simulink model "ddddddddd"  (R2020a)
settings: Solver=VariableStepAuto  StartTime=0.0  StopTime=1  RelTol=1e-3
libraries: powerlib x19, powerlib_meascontrol x4
settings Model: Creator=hp  LastModifiedBy=hp

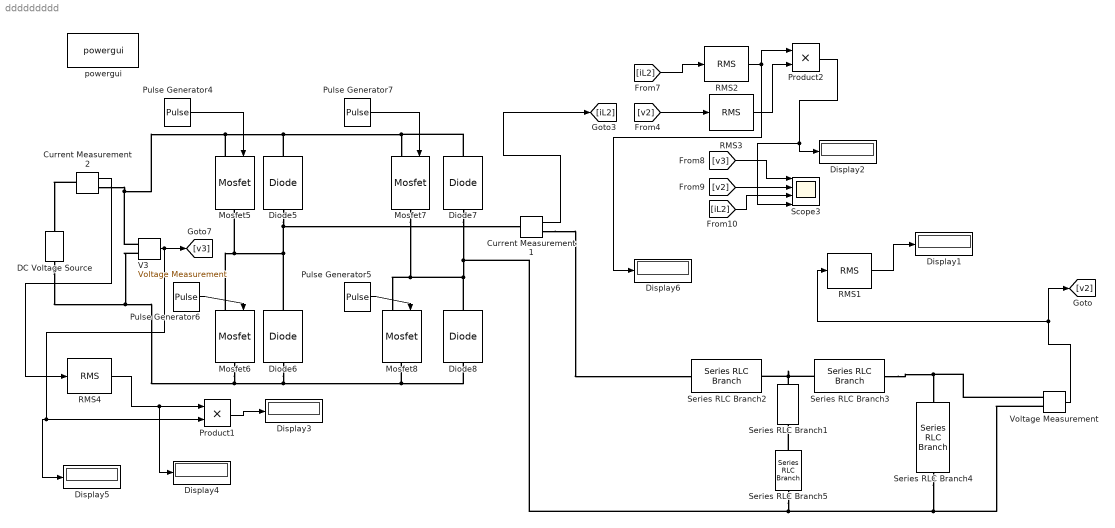
== system ddddddddd ==
  Current Measurement1 : powerlib/Measurements/Current Measurement  PhasorSimulation=off  OutputType=Complex  PSBequivalent=0
  Current Measurement2 : powerlib/Measurements/Current Measurement  PhasorSimulation=off  OutputType=Complex  PSBequivalent=0
  DC Voltage Source : powerlib/Electrical Sources/DC Voltage Source  Amplitude=900  Measurements=None
  Diode{5..8} (4 alike) : powerlib/Power Electronics/Diode  Ron=0.001  Lon=0  Vf=0.8  IC=0  UseSnubber=0  Rs=500  Cs=250e-9  Measurements=off
  Display{1..6} (6 alike) : Display
  Mosfet{5..8} (4 alike) : powerlib/Power Electronics/Mosfet  Ron=0.1  Lon=0  Rd=0.01  Vfd=0  IC=0  Rs=1e5  Cs=inf  Measurements=off
  Product1 : Product
  Product2 : Product
  Pulse Generator4 : DiscretePulseGenerator  PulseType=Time based  Period=1/(10000)  PulseWidth=50  PhaseDelay=0/(360*5000)
  Pulse Generator5 : DiscretePulseGenerator  PulseType=Time based  Period=1/(10000)  PulseWidth=50  PhaseDelay=0/(360*5000)
  Pulse Generator6 : DiscretePulseGenerator  PulseType=Time based  Period=1/(10000)  PulseWidth=50  PhaseDelay=180/(360*10000)
  Pulse Generator7 : DiscretePulseGenerator  PulseType=Time based  Period=1/(10000)  PulseWidth=50  PhaseDelay=180/(360*10000)
  RMS{1..4} (4 alike) : powerlib_meascontrol/Measurements/RMS  TrueRMS=on  Freq=60  RMSInit=120  Ts=0
  Scope3 : Scope  NumInputPorts=4
  Series RLC Branch1 : powerlib/Elements/Series RLC Branch  LConnTagsString=__new0  RConnTagsString=__new0  BranchType=C  Resistance=181  Inductance=1e-3  SetiL0=off  InitialCurrent=0  Capacitance=1.5e-5  Setx0=off  InitialVoltage=0  Measurements=None
  Series RLC Branch2 : powerlib/Elements/Series RLC Branch  LConnTagsString=__new0  RConnTagsString=__new0  BranchType=RL  Resistance=1e-3  Inductance=10e-4  SetiL0=off  InitialCurrent=0  Capacitance=1e-6  Setx0=off  InitialVoltage=0  Measurements=None
  Series RLC Branch3 : powerlib/Elements/Series RLC Branch  LConnTagsString=__new0  RConnTagsString=__new0  BranchType=RL  Resistance=1e-3  Inductance=11e-4  SetiL0=off  InitialCurrent=0  Capacitance=1e-6  Setx0=off  InitialVoltage=0  Measurements=None
  Series RLC Branch4 : powerlib/Elements/Series RLC Branch  LConnTagsString=__new0  RConnTagsString=__new0  BranchType=R  Resistance=181  Inductance=1e-3  SetiL0=off  InitialCurrent=0  Capacitance=1e-6  Setx0=off  InitialVoltage=0  Measurements=None
  Series RLC Branch5 : powerlib/Elements/Series RLC Branch  LConnTagsString=__new0  RConnTagsString=__new0  BranchType=R  Resistance=22.15  Inductance=1e-3  SetiL0=off  InitialCurrent=0  Capacitance=1e-6  Setx0=off  InitialVoltage=0  Measurements=None
  V3 : powerlib/Measurements/Voltage Measurement  PhasorSimulation=off  OutputType=Complex  PSBequivalent=0
  Voltage Measurement : powerlib/Measurements/Voltage Measurement  PhasorSimulation=off  OutputType=Complex  PSBequivalent=0
  powergui : powerlib/powergui  Priority=1  SimulationMode=Discrete  SampleTime=50e-8  frequency=60  Iterations=50  frequencyindice=0  Pbase=100e6  ErrMax=1e-4  UnitsV=kV  UnitsW=MW  buscounter=0  FunctionMessages=off  echomessages=off  EnableUseOfTLC=off  CurrentSourceSwitches=off  DisableSnubberDevices=off  DisableRonSwitches=off  DisableVfSwitches=off  DisplayEquations=off  AutomaticDiscreteSolvers=off  SolverType=Tustin/Backward Euler (TBE)  Interpol=off  ExternalGateDelay=off  methode=off  Ts=100  x0status=blocks  SPID=on  SwTol=0  HookPort=off  NonlinearTolerance=1e-4  nMaxIteration=100  ContinueOnMaxIteration=off  RestoreLinks=warning  ResistiveCurrentMeasurement=off  Frange=[0:2:500]  Ylog=off  Xlog=on  ShowGrid=off  save=off  variable=ZData  structure=0  ZoomFFT=off  StartTime=0.0  cycles=1  DisplayStyle=1  fundamental=60  FreqAxis=off  MaxFrequency=1000  frequencyindicesteady=1  RmsSteady=1  display=off
  wires:
  [iL2] -> RMS2/1
  [iL2] -> Scope3/3
  RMS2/1 -> Display6/1, Product2/1
  RMS3/1 -> Product2/2
  [v2] -> RMS3/1
  Pulse Generator5/1 -> Mosfet8/1
  [v3] -> Scope3/1
  Pulse Generator4/1 -> Mosfet5/1
  Pulse Generator6/1 -> Mosfet6/1
  Current Measurement1/1 -> [iL2]
  Product2/1 -> Display2/1, Scope3/4
  [v2] -> Scope3/2
  Pulse Generator7/1 -> Mosfet7/1
  Voltage Measurement/1 -> RMS1/1, [v2]
  RMS1/1 -> Display1/1
  Current Measurement2/1 -> RMS4/1
  RMS4/1 -> Display4/1, Product1/1
  V3/1 -> Product1/2, Display5/1, [v3]
  Product1/1 -> Display3/1
  connections:
  Mosfet7/RConn1 -- Diode8/RConn1 -- Diode7/LConn1 -- Voltage Measurement/LConn2 -- Series RLC Branch4/RConn1 -- Series RLC Branch5/RConn1 -- Mosfet8/LConn1
  V3/LConn1 -- Current Measurement2/RConn1 -- Diode5/RConn1 -- Diode7/RConn1 -- Mosfet7/LConn1 -- Mosfet5/LConn1
  Mosfet6/LConn1 -- Mosfet5/RConn1 -- Diode6/RConn1 -- Diode5/LConn1 -- Current Measurement1/LConn1
  Mosfet6/RConn1 -- Diode8/LConn1 -- Mosfet8/RConn1 -- Diode6/LConn1 -- V3/LConn2 -- DC Voltage Source/LConn1
  Voltage Measurement/LConn1 -- Series RLC Branch3/RConn1 -- Series RLC Branch4/LConn1
  Series RLC Branch1/LConn1 -- Series RLC Branch3/LConn1 -- Series RLC Branch2/RConn1
  Series RLC Branch5/LConn1 -- Series RLC Branch1/RConn1
  Current Measurement1/RConn1 -- Series RLC Branch2/LConn1
  Current Measurement2/LConn1 -- DC Voltage Source/RConn1
